simulink model "Ebora_Zandro_Zevastien_Zyn_A_SIMULINK_5"  (R2023b)
settings: Solver=VariableStepAuto  StartTime=0.0  StopTime=20  RelTol=1e-3
values from neighbouring files (symbols this model uses):
  F_den = [1 2 3 4 5 6 7 1]    [Ebora_Zandro_Zevastien_Zyn_A_MATLAB_5_and_6.m]
  F_num = [8 7 6 5 4 3 2]    [Ebora_Zandro_Zevastien_Zyn_A_MATLAB_5_and_6.m]
settings Model: Creator=Troy  LastModifiedBy=Troy

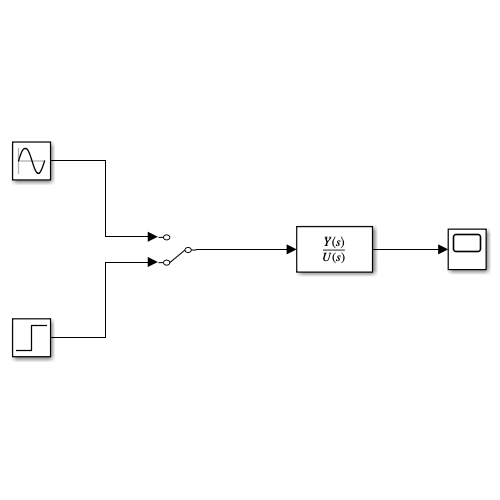
[thumbnail: Simulink's stored preview of the top-level diagram]
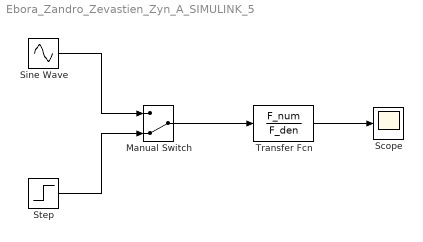
== system Ebora_Zandro_Zevastien_Zyn_A_SIMULINK_5 ==
  Manual Switch : ManualSwitch  CurrentSetting=0
  Scope : Scope
  Sine Wave : Sin  SampleTime=0
  Step : Step  Time=0  SampleTime=0
  Transfer Fcn : TransferFcn  Numerator=F_num  Denominator=F_den
  wires:
  Sine Wave/1 -> Manual Switch/1
  Step/1 -> Manual Switch/2
  Manual Switch/1 -> Transfer Fcn/1
  Transfer Fcn/1 -> Scope/1
